simulink model "Design_model"  (R2025b)
settings: Solver=FixedStepAuto  StartTime=0.0  StopTime=Tf  FixedStep=Tsample  RelTol=1e-3
values from neighbouring files (symbols this model uses):
  Kd = (2*zeta*Wn - Pm) / (Km * Pm)    [Designation_matlab.m]
  Km = 10.7936 / 10.7132    (= 1.00750476048)    [Designation_mat.m]    (also in Designation_matlab.m = 1301)
  Kp = Wn^2 / (Km * Pm)    (= 0.106517797472)    [Designation_matlab.m]
  Time_const = 1 / 10.7132    (= 0.0933427920696)    [Designation_mat.m]
settings Model: Creator=GILBERT  LastModifiedBy=GILBERT

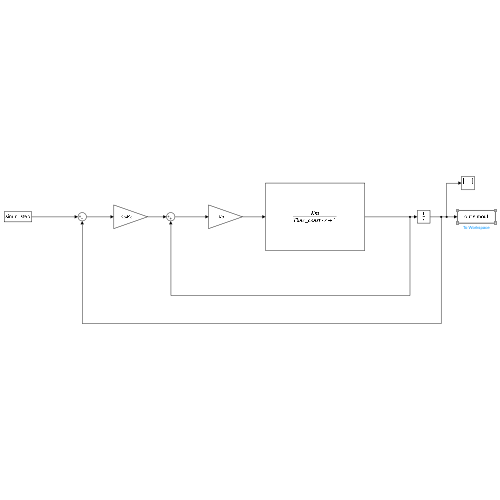
[thumbnail: Simulink's stored preview of the top-level diagram]
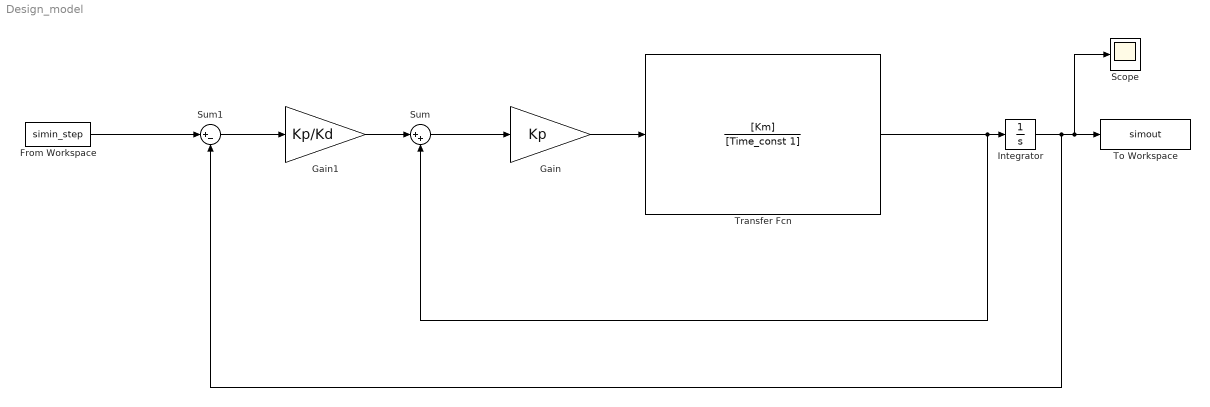
== system Design_model ==
  From Workspace : FromWorkspace  VariableName=simin_step
  Gain : Gain  Gain=Kp
  Gain1 : Gain  Gain=Kp/Kd
  Integrator : Integrator
  Scope : Scope
      settings: ActiveDisplayYMinimum=-6.8987550060025909E+303  ActiveDisplayYMaximum=9.00330787681435E+303
  Sum : Sum  Inputs=|++
  Sum1 : Sum  Inputs=|+-
  To Workspace : ToWorkspace  VariableName=simout  SaveFormat=Timeseries  SampleTime=-1
  Transfer Fcn : TransferFcn  Numerator=[Km]  Denominator=[Time_const 1]
  wires:
  Transfer Fcn/1 -> Integrator/1, Sum/2
  Sum/1 -> Gain/1
  Gain/1 -> Transfer Fcn/1
  Integrator/1 -> Sum1/2, Scope/1, To Workspace/1
  Gain1/1 -> Sum/1
  From Workspace/1 -> Sum1/1
  Sum1/1 -> Gain1/1
